simulink model "convolution_2D"  (R2024b)
settings: Solver=FixedStepDiscrete  StartTime=0.0  StopTime=100  RelTol=1e-3
InitFcn:
  | % Define a random matrix size between 3 and 10
  | n =4;
  | 
  | fprintf('Size of matrix A: n = %d\n', n);
libraries: visionhdlio x1, hdlsllib x1, visionhdlutilities x1
settings Model: DataTypeOverride=Off  Creator=valen  LastModifiedBy=valen
settings SolverCC: AlgebraicLoopSolver=TrustRegion
settings DataIOCC: LimitDataPoints=on  SaveOutput=off  SaveTime=off
settings OptimizationCC: BlockReduction=off  ConditionallyExecuteInputs=off  DefaultParameterBehavior=Inlined  LifeSpan=inf
settings DebuggingCC: AlgebraicLoopMsg=error  SingleTaskRateTransMsg=error  UnconnectedInputMsg=warning  UnconnectedOutputMsg=warning  UnconnectedLineMsg=warning  AllowSymbolicDim=off  StrictBusMsg=ErrorOnBusTreatedAsVector  SFUnexpectedBacktrackingDiag=warning  SFNoUnconditionalDefaultTransitionDiag=warning  SFExecutionAtInitializationDiag=none  ArithmeticOperatorsInVariantConditions=warning
settings HardwareCC: ProdBitPerPointer=32  ProdBitPerSizeT=32  ProdBitPerPtrDiffT=32  ProdLargestAtomicFloat=None  ProdIntDivRoundTo=Undefined  ProdEndianess=Unspecified  ProdWordSize=32  ProdHWDeviceType=ASIC/FPGA->ASIC/FPGA  ProdEqTarget=off
settings ModelReferenceCC: EnableRefExpFcnMdlSchedulingChecks=on
settings SFSimCC: SimUseLocalCustomCode=off  CustomCodeUndefinedFunction=UseInterfaceOnly
settings RTWCC: RTWUseLocalCustomCode=off  GPUComputeCapability=3.5
settings CodeAppCC: StateflowObjectComments=on
settings GRTTargetCC: TargetLangStandard=C89/C90 (ANSI)
settings ConfigComp: CovScope=ReferencedModels  CovMetricSettings=dw  CovSaveCumulativeToWorkspaceVar=on  CovSaveSingleToWorkspaceVar=on  CovExternalEMLEnable=off  CovSFcnEnable=off

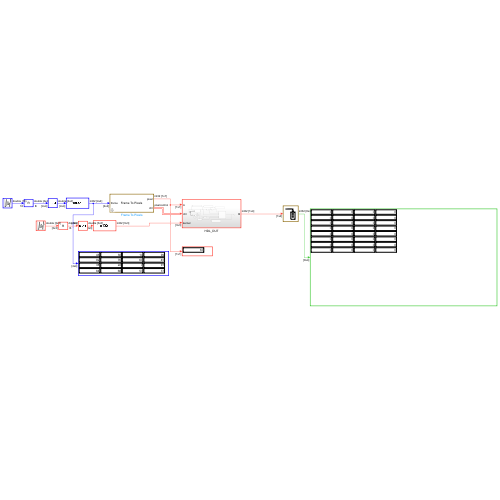
[thumbnail: Simulink's stored preview of the top-level diagram]
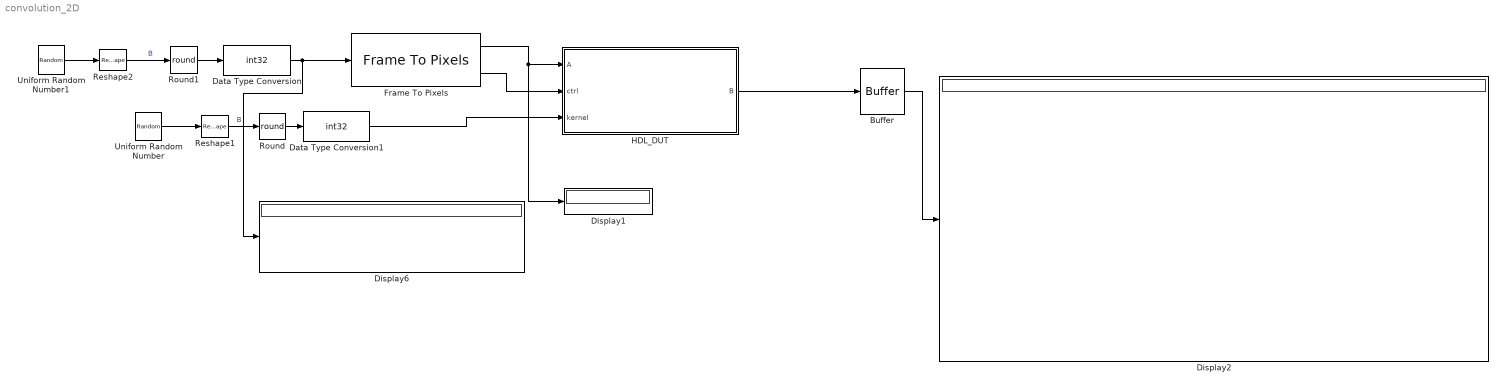
== system convolution_2D ==
  Buffer : Buffer  N=2*n  OutputFrames=off
  Data Type Conversion : DataTypeConversion  OutDataTypeStr=int32  SaturateOnIntegerOverflow=off  RndMeth=Floor
  Data Type Conversion1 : DataTypeConversion  OutDataTypeStr=int32  SaturateOnIntegerOverflow=off  RndMeth=Floor
  Display1 : Display
  Display2 : Display
  Display6 : Display
  Frame To Pixels : visionhdlio/Frame To Pixels  NumComponents=1  NumPixels=1  VideoFormat=Custom  ActivePixelsPerLine=n  ActiveVideoLines=n  TotalPixelsPerLine=n  TotalVideoLines=n  StartingActiveLine=1  FrontPorch=0  SampleTime=0  VideoFormatCache=Custom  ActivePixelsPerLineCache=n  ActiveVideoLinesCache=n  TotalPixelsPerLineCache=n  TotalVideoLinesCache=n  StartingActiveLineCache=1  FrontPorchCache=0
  HDL_DUT : Subsystem
  Reshape1 : Reshape  OutputDimensionality=Customize  OutputDimensions=[3,3]
  Reshape2 : Reshape  OutputDimensionality=Customize  OutputDimensions=[n,n]
  Round : Rounding  Operator=round
  Round1 : Rounding  Operator=round
  Uniform Random Number : UniformRandomNumber  Minimum=0  Maximum=100  Seed=randi([0,100],3)  SampleTime=0.00625
  Uniform Random Number1 : UniformRandomNumber  Minimum=0  Maximum=100  Seed=[1:n*n]  SampleTime=0.1
  wires:
  Round1/1 -> Data Type Conversion/1
  HDL_DUT/1(B) -> Buffer/1
  Reshape1/1 -> Round/1  "B"
  Uniform Random Number/1 -> Reshape1/1
  Round/1 -> Data Type Conversion1/1
  Buffer/1 -> Display2/1
  Uniform Random Number1/1 -> Reshape2/1
  Reshape2/1 -> Round1/1  "B"
  Data Type Conversion/1 -> Display6/1, Frame To Pixels/1
  Frame To Pixels/1 -> Display1/1, HDL_DUT/1(A)
  Frame To Pixels/2 -> HDL_DUT/2(ctrl)
  Data Type Conversion1/1 -> HDL_DUT/3(kernel)

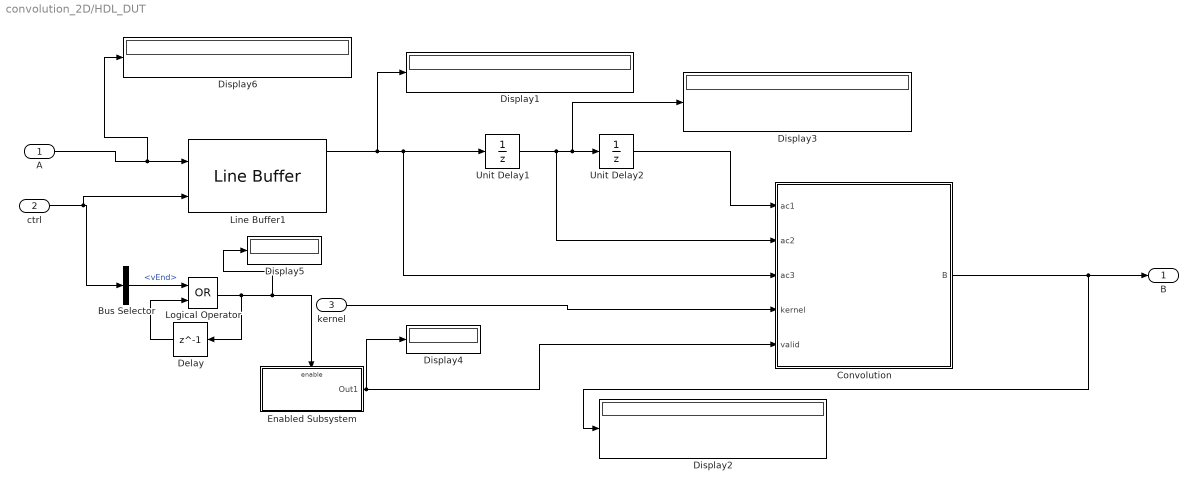
== system convolution_2D/HDL_DUT ==
  A : Inport
  ctrl : Inport  Port=2
  kernel : Inport  Port=3
  Bus Selector : BusSelector  OutputSignals=vEnd
  Convolution : MATLAB Function  TreatAsAtomicUnit=on
  Delay : Delay  DelayLength=1  InitialCondition=0
  Display{1..6} (6 alike) : Display
  Enabled Subsystem : Subsystem  TreatAsAtomicUnit=on
  Line Buffer1 : visionhdlutilities/Line Buffer  NeighborhoodSize=[n,1]  PaddingMethod=Constant  PaddingValue=0  LineBufferSize=16  SimulateUsing=Code generation
  Logical Operator : Logic  Operator=OR  AllPortsSameDT=off  OutDataTypeStr=boolean
  Unit Delay1 : UnitDelay  InputProcessing=Columns as channels (frame based)  SampleTime=-1  HasFrameUpgradeWarning=on
  Unit Delay2 : UnitDelay  InputProcessing=Columns as channels (frame based)  SampleTime=-1  HasFrameUpgradeWarning=on
  B : Outport  VectorParamsAs1DForOutWhenUnconnected=off
  wires:
  kernel/1 -> Convolution/4(kernel)
  Convolution/1(B) -> Display2/1, B/1
  Unit Delay1/1 -> Convolution/2(ac2), Display3/1, Unit Delay2/1
  Unit Delay2/1 -> Convolution/1(ac1)
  Line Buffer1/1 -> Display1/1, Convolution/3(ac3), Unit Delay1/1
  A/1 -> Display6/1, Line Buffer1/1
  ctrl/1 -> Line Buffer1/2, Bus Selector/1
  Enabled Subsystem/1(Out1) -> Display4/1, Convolution/5(valid)
  Bus Selector/1 -> Logical Operator/1  "<vEnd>"
  Logical Operator/1 -> Delay/1, Display5/1, Enabled Subsystem/Enable
  Delay/1 -> Logical Operator/2

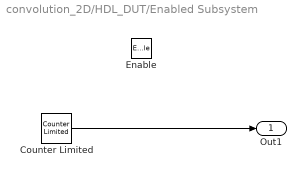
== system convolution_2D/HDL_DUT/Enabled Subsystem ==
  Enable : EnablePort
  Counter Limited : hdlsllib/Sources/Counter Limited  uplimit=9  tsamp=-1
  Out1 : Outport
  wires:
  Counter Limited/1 -> Out1/1

== matlab function convolution_2D/HDL_DUT/Convolution ==
  data: ac1 input; ac2 input; ac3 input; B output; kernel input; valid input
function B = fcn(ac1,ac2,ac3,kernel, valid)
   m=length(ac2);
   B=zeros(1,m,'like',ac2);
    if (valid<=m && valid>0)
        kernel_size=length(kernel);
        kernel_rad = floor(kernel_size / 2);
        for y=1:m
            sum=cast(0,'int32');
            for i=-kernel_rad:kernel_rad
                for j=-kernel_rad:kernel_rad
                    value=cast(0,'int32');
                    if (i == -1 && valid<2) % Ligne ac1 invalide
                        value = cast(0, 'int32');
                    elseif (i == 1 && valid>m-1) % Ligne ac3 invalide
                        value = cast(0, 'int32');
                    else
                        if (y+j<=0||y+j>m)
                             value = cast(0, 'int32');
                        elseif (i>0)
                            value = ac3(y+j);
                        elseif (i<0)
                            value= ac1(y+j);
                        else
                            value =ac2(y+j);
                        end
                    end
                    sum=sum+value*kernel(i+kernel_rad+1,j+kernel_rad+1);
                end
            end
            B(y)=sum;
        end
    end
end
